simulink model "comparcion"  (R2019a)
settings: Solver=VariableStepAuto  StartTime=0.0  StopTime=10  MaxStep=1e-4  RelTol=1e-3
values from neighbouring files (symbols this model uses):
  alfa_cu = 3.9 * 10^(-3)    (= 0.0039)    [Datos.m]
  bl = 0    [Datos.m]
  bm = 1.5 * 10^(-5)    (= 1.5e-05)    [Datos.m]
  Cts = 0.818    [Datos.m]
  Jl = 0.2520    (= 0.252)    [Datos.m]
  Jm = 3.1 * 10^(-6)    (= 3.1e-06)    [Datos.m]
  lambda_m_r = 0.01546    [Datos.m]
  Ld = 6.6e-3    (= 0.0066)    [Datos.m]
  Lq = 5.8e-3    (= 0.0058)    [Datos.m]
  Pp = 3    [Datos.m]
  r = 314.3008    [Datos.m]
  Rts_amb = 146.7    [Datos.m]
undefined symbols (not defined in the file or in its folder): magnitude, sigbuilder_block
settings Model: OrderedModelArguments=off  Creator=renzo  LastModifiedBy=renzo

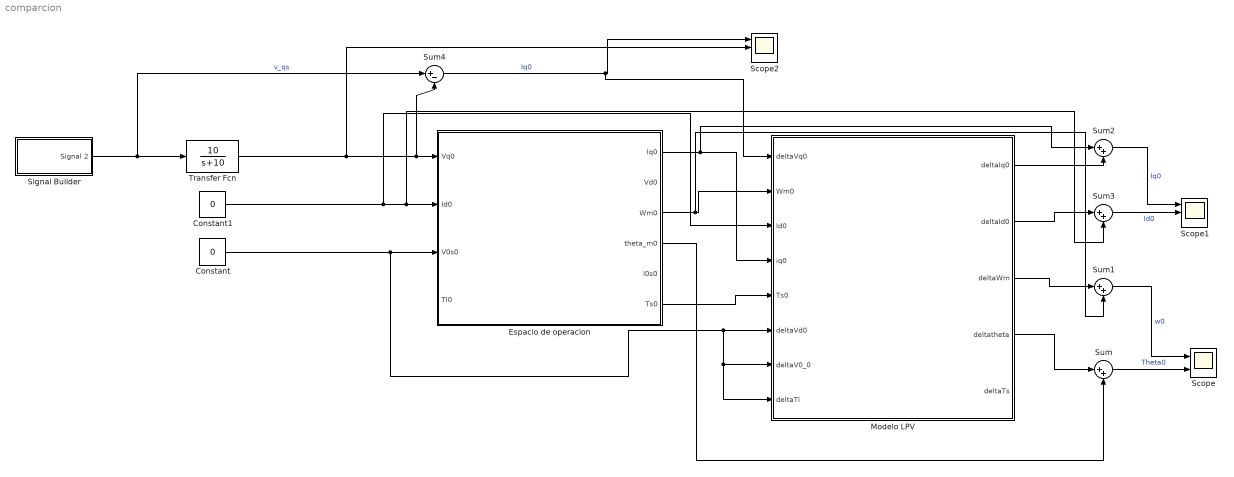
== system comparcion ==
  Constant : Constant  Value=0
  Constant1 : Constant  Value=0
  "Espacio de operacion " : Subsystem
  "Modelo LPV " : Subsystem
  Scope : Scope  NumInputPorts=2
  Scope1 : Scope  NumInputPorts=3
  Scope2 : Scope  NumInputPorts=3
  Signal Builder : Subsystem  Tag=STV Subsys  LoadFcn=sigbuilder_block('load');  StartFcn=sigbuilder_block('start');  StopFcn=sigbuilder_block('stop');  ClipboardFcn=sigbuilder_block('clipboard');  mask(Sigbuilder block){tuvar=[0:10]}
      mask help: Simulink:masks:SigbuilderBlock_MD
      mask init:
      | if ~strcmp(get_param(bdroot(gcbh),'SimulationStatus'),'stopped') tuvar = sigbuilder_block('maskInit'); end
      settings: CopyFcn=sigbuilder_block('copy');  DeleteFcn=sigbuilder_block('delete');  ModelCloseFcn=sigbuilder_block('modelClose');  PreSaveFcn=sigbuilder_block('preSave');  PauseFcn=sigbuilder_block('pause');  ContinueFcn=sigbuilder_block('continue');  NameChangeFcn=sigbuilder_block('namechange');  OpenFcn=sigbuilder_block('open',[437.6 153 550.4 359.25 ]);  CloseFcn=sigbuilder_block('close');
      mask Display: plot(0, 0, 100, 100,[2, 2, 32, 32, 2], [68, 8, 8, 68, 68],[32, 2], [38, 38], [32, 19, 2],[53, 60, 44], [32, 17, 17, 2],[16, 16, 31, 31]);txt = getActiveGroup(gcbh);text(2, 100, txt,'verticalAlignment', 'top');
  Sum{,1..3} (4 alike) : Sum  Inputs=|++
  Sum4 : Sum  Inputs=|+-
  Transfer Fcn : TransferFcn  Numerator=[10]  Denominator=[1 10]
  wires:
  Sum2/1 -> Scope1/1  "Iq0"
  Sum3/1 -> Scope1/2  "Id0"
  Transfer Fcn/1 -> Scope2/2, "Espacio de operacion "/1(Vq0), Sum4/2
  Sum4/1 -> "Modelo LPV "/1(deltaVq0), Scope2/1  "Iq0"
  Constant1/1 -> "Modelo LPV "/3(Id0), Sum3/2, "Espacio de operacion "/2(Id0)
  Constant/1 -> "Modelo LPV "/8(deltaTl), "Modelo LPV "/7("deltaV0_0 "), "Modelo LPV "/6("deltaVd0 "), "Espacio de operacion "/3(V0s0)
  "Espacio de operacion "/1(Iq0) -> Sum2/1, "Modelo LPV "/4(iq0)
  "Espacio de operacion "/3(Wm0) -> Sum1/2, "Modelo LPV "/2(Wm0)
  "Modelo LPV "/1("deltaIq0 ") -> Sum2/2
  "Modelo LPV "/2(deltaId0) -> Sum3/1
  "Modelo LPV "/3(deltaWm) -> Sum1/1
  "Espacio de operacion "/4(theta_m0) -> Sum/2
  "Modelo LPV "/4(deltatheta) -> Sum/1
  Sum1/1 -> Scope/1  "w0"
  Sum/1 -> Scope/2  "Theta0"
  Signal Builder/1(Signal 2) -> Sum4/1, Transfer Fcn/1  "v_qs"
  "Espacio de operacion "/6(Ts0) -> "Modelo LPV "/5(Ts0)

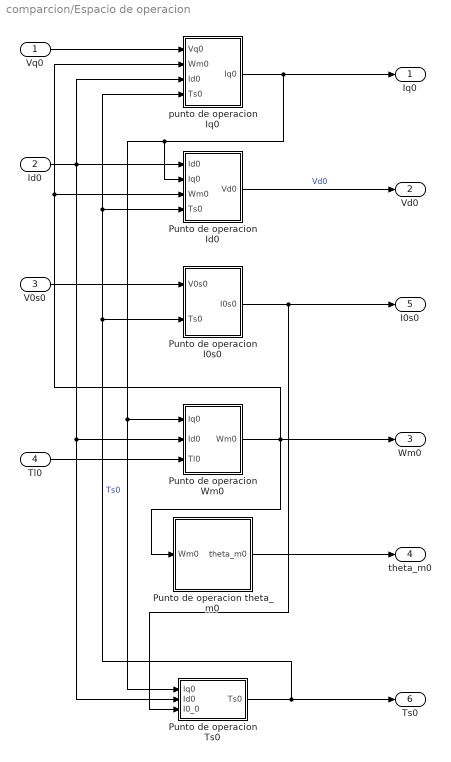
== system comparcion/Espacio de operacion  ==
  Vq0 : Inport
  Id0 : Inport  Port=2
  V0s0 : Inport  Port=3
  "Tl0 " : Inport  Port=4
  Punto de operacion I0s0 : Subsystem
  Punto de operacion Id0 : Subsystem
  Punto de operacion Ts0 : Subsystem
  Punto de operacion Wm0 : Subsystem
  Punto de operacion theta_m0 : Subsystem
  "punto de operacion Iq0 " : Subsystem
  Iq0 : Outport
  Vd0 : Outport  Port=2
  Wm0 : Outport  Port=3
  theta_m0 : Outport  Port=4
  I0s0 : Outport  Port=5
  Ts0 : Outport  Port=6
  wires:
  Punto de operacion Wm0/1("Wm0 ") -> Wm0/1, Punto de operacion Id0/3(Wm0), "punto de operacion Iq0 "/2("Wm0 "), Punto de operacion theta_m0/1(Wm0)
  Punto de operacion Ts0/1(Ts0) -> Ts0/1, Punto de operacion Id0/4("Ts0 "), "punto de operacion Iq0 "/4(Ts0), Punto de operacion I0s0/2("Ts0 ")  "Ts0"
  Punto de operacion I0s0/1("I0s0 ") -> Punto de operacion Ts0/3("I0_0 "), I0s0/1
  "punto de operacion Iq0 "/1("Iq0 ") -> Punto de operacion Id0/2("Iq0 "), Punto de operacion Wm0/1(Iq0), Punto de operacion Ts0/1(Iq0), Iq0/1
  Punto de operacion theta_m0/1("theta_m0 ") -> theta_m0/1
  Punto de operacion Id0/1("Vd0 ") -> Vd0/1  "Vd0"
  V0s0/1 -> Punto de operacion I0s0/1("V0s0 ")
  Vq0/1 -> "punto de operacion Iq0 "/1(Vq0)
  "Tl0 "/1 -> Punto de operacion Wm0/3("Tl0 ")
  Id0/1 -> Punto de operacion Ts0/2(Id0), Punto de operacion Wm0/2("Id0 "), "punto de operacion Iq0 "/3("Id0 "), Punto de operacion Id0/1("Id0 ")

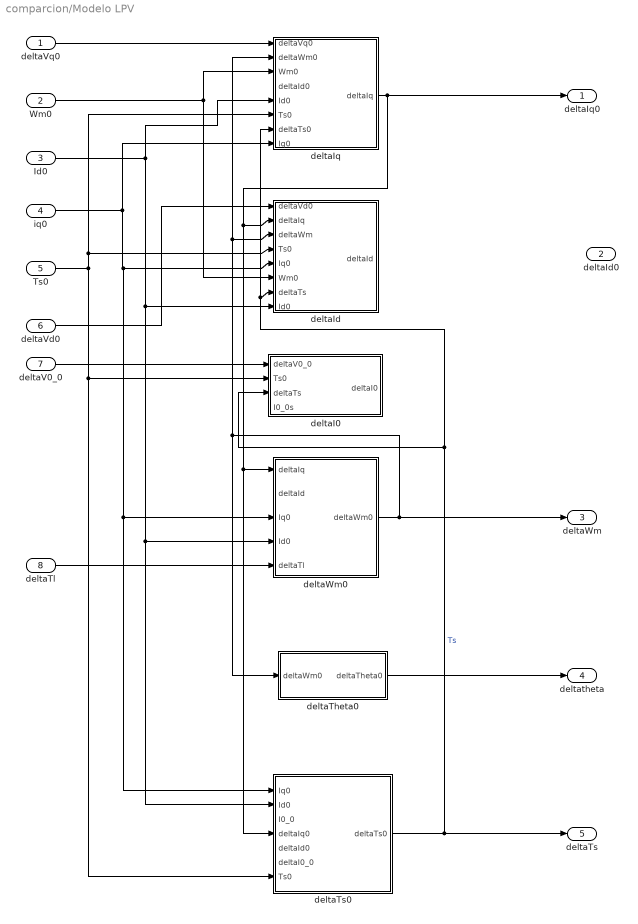
== system comparcion/Modelo LPV  ==
  deltaVq0 : Inport
  Wm0 : Inport  Port=2
  Id0 : Inport  Port=3
  iq0 : Inport  Port=4
  Ts0 : Inport  Port=5
  "deltaVd0 " : Inport  Port=6
  "deltaV0_0 " : Inport  Port=7
  deltaTl : Inport  Port=8
  deltaI0 : Subsystem
  deltaId : Subsystem
  deltaIq : Subsystem
  deltaTheta0 : Subsystem
  "deltaTs0 " : Subsystem
  deltaWm0 : Subsystem
  "deltaIq0 " : Outport
  deltaId0 : Outport  Port=2
  deltaWm : Outport  Port=3
  deltatheta : Outport  Port=4
  deltaTs : Outport  Port=5
  wires:
  "deltaTs0 "/1(deltaTs0) -> deltaTs/1, deltaIq/7("deltaTs0 "), deltaId/7(deltaTs), deltaI0/3(deltaTs)  "Ts"
  Ts0/1 -> "deltaTs0 "/7("Ts0 "), deltaI0/2("Ts0 "), deltaId/4("Ts0 "), deltaIq/6("Ts0 ")
  deltaVq0/1 -> deltaIq/1(deltaVq0)
  deltaWm0/1("deltaWm0 ") -> deltaWm/1, deltaTheta0/1("deltaWm0 "), deltaIq/2("deltaWm0 "), deltaId/3("deltaWm ")
  Wm0/1 -> deltaId/6(Wm0), deltaIq/3(Wm0)
  Id0/1 -> deltaId/8(Id0), "deltaTs0 "/2(Id0), deltaWm0/4("Id0 "), deltaIq/5(Id0)
  iq0/1 -> "deltaTs0 "/1("Iq0 "), deltaWm0/3("Iq0 "), deltaId/5(Iq0), deltaIq/8(Iq0)
  deltaIq/1(deltaIq) -> deltaWm0/1(deltaIq), "deltaTs0 "/4("deltaIq0 "), deltaId/2("deltaIq "), "deltaIq0 "/1
  "deltaVd0 "/1 -> deltaId/1(deltaVd0)
  "deltaV0_0 "/1 -> deltaI0/1(deltaV0_0)
  deltaTl/1 -> deltaWm0/5(deltaTl)
  deltaTheta0/1("deltaTheta0 ") -> deltatheta/1

== system comparcion/Signal Builder ==
  Demux : Demux  Tag=STV Demux  Outputs=1
  FromWs : FromWorkspace  Tag=STV FromWs  VariableName=tuvar  SampleTime=0
      SigBuilderData=|
      | common.afterFinalStr = 'Extrapolate'
      | common.sampleTime = 0
      | dataSet.timeRange = [0 10]
      | dataSet.name = 'Group 1'
      | sbobj.Groups.Name = 'Group 1'
      | sbobj.Groups.Signals.Name = 'Signal 2'
      | sbobj.Groups.Signals.XData = [0 1 1 10]
      | sbobj.Groups.Signals.YData = [0 0 1 1]
  Signal 2 : Outport  Tag=STV Outport
  wires:
  FromWs/1 -> Demux/1
  Demux/1 -> Signal 2/1

== system comparcion/Espacio de operacion /Punto de operacion I0s0 ==
  "V0s0 " : Inport
  "Ts0 " : Inport  Port=2
  Divide : Product  Inputs=*/
  Rs(t) : Subsystem
  "I0s0 " : Outport
  wires:
  "V0s0 "/1 -> Divide/1
  "Ts0 "/1 -> Rs(t)/1(Ts)
  Rs(t)/1(Rs) -> Divide/2
  Divide/1 -> "I0s0 "/1

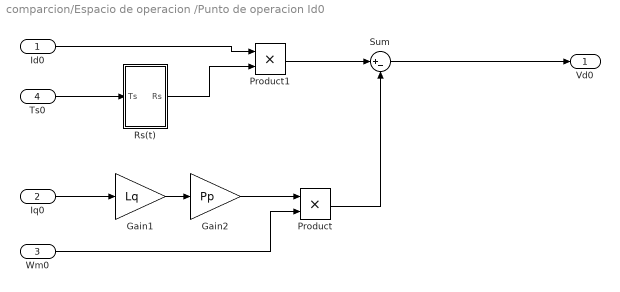
== system comparcion/Espacio de operacion /Punto de operacion Id0 ==
  "Id0 " : Inport
  "Iq0 " : Inport  Port=2
  Wm0 : Inport  Port=3
  "Ts0 " : Inport  Port=4
  Gain1 : Gain  Gain=Lq
  Gain2 : Gain  Gain=Pp
  Product : Product
  Product1 : Product
  Rs(t) : Subsystem
  Sum : Sum  Inputs=|+-
  "Vd0 " : Outport
  wires:
  "Iq0 "/1 -> Gain1/1
  Gain2/1 -> Product/1
  Gain1/1 -> Gain2/1
  Wm0/1 -> Product/2
  Product/1 -> Sum/2
  "Ts0 "/1 -> Rs(t)/1(Ts)
  Sum/1 -> "Vd0 "/1
  Rs(t)/1(Rs) -> Product1/2
  "Id0 "/1 -> Product1/1
  Product1/1 -> Sum/1

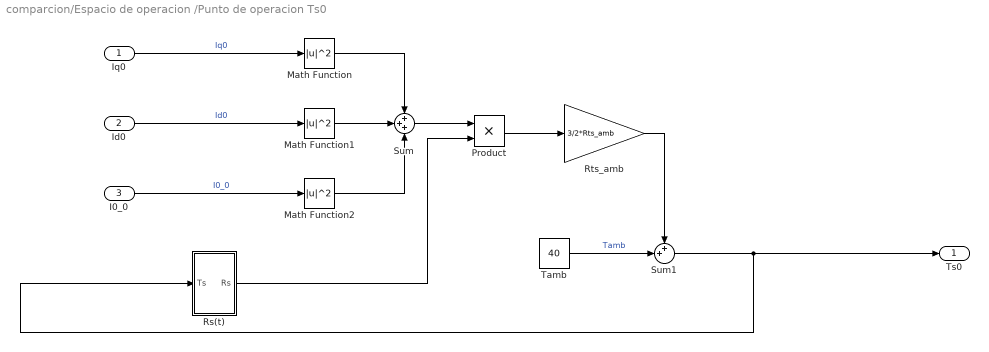
== system comparcion/Espacio de operacion /Punto de operacion Ts0 ==
  Iq0 : Inport
  Id0 : Inport  Port=2
  "I0_0 " : Inport  Port=3
  Math Function : Math  Operator=magnitude^2  SaturateOnIntegerOverflow=on
  Math Function1 : Math  Operator=magnitude^2  SaturateOnIntegerOverflow=on
  Math Function2 : Math  Operator=magnitude^2  SaturateOnIntegerOverflow=on
  Product : Product
  Rs(t) : Subsystem
  Rts_amb : Gain  Gain=3/2*Rts_amb
  Sum : Sum  Inputs=3
  Sum1 : Sum  Inputs=++|
  Tamb : Constant  Value=40
  Ts0 : Outport  VectorParamsAs1DForOutWhenUnconnected=on
  wires:
  Iq0/1 -> Math Function/1  "Iq0"
  Id0/1 -> Math Function1/1  "Id0"
  "I0_0 "/1 -> Math Function2/1  "I0_0"
  Math Function1/1 -> Sum/2
  Math Function/1 -> Sum/1
  Math Function2/1 -> Sum/3
  Sum/1 -> Product/1
  Product/1 -> Rts_amb/1
  Tamb/1 -> Sum1/2  "Tamb"
  Sum1/1 -> Ts0/1, Rs(t)/1(Ts)
  Rs(t)/1(Rs) -> Product/2
  Rts_amb/1 -> Sum1/1

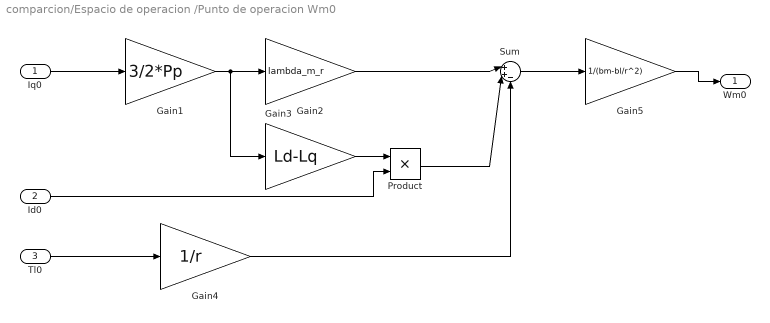
== system comparcion/Espacio de operacion /Punto de operacion Wm0 ==
  Iq0 : Inport
  "Id0 " : Inport  Port=2
  "Tl0 " : Inport  Port=3
  Gain1 : Gain  Gain=3/2*Pp
  Gain2 : Gain  Gain=lambda_m_r
  Gain3 : Gain  Gain=Ld-Lq
  Gain4 : Gain  Gain=1/r
  Gain5 : Gain  Gain=1/(bm-bl/r^2)
  Product : Product
  Sum : Sum  Inputs=|++-
  "Wm0 " : Outport
  wires:
  Iq0/1 -> Gain1/1
  Gain1/1 -> Gain3/1, Gain2/1
  Gain2/1 -> Sum/1
  Gain3/1 -> Product/1
  "Id0 "/1 -> Product/2
  Product/1 -> Sum/2
  "Tl0 "/1 -> Gain4/1
  Gain4/1 -> Sum/3
  Sum/1 -> Gain5/1
  Gain5/1 -> "Wm0 "/1

== system comparcion/Espacio de operacion /Punto de operacion theta_m0 ==
  Wm0 : Inport
  Integrator : Integrator
  "theta_m0 " : Outport
  wires:
  Wm0/1 -> Integrator/1
  Integrator/1 -> "theta_m0 "/1

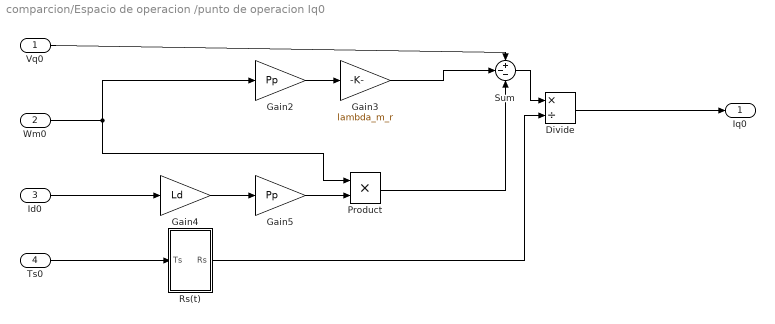
== system comparcion/Espacio de operacion /punto de operacion Iq0  ==
  Vq0 : Inport
  "Wm0 " : Inport  Port=2
  "Id0 " : Inport  Port=3
  Ts0 : Inport  Port=4
  Divide : Product  Inputs=*/
  Gain2 : Gain  Gain=Pp
  Gain3 : Gain  Gain=lambda_m_r
  Gain4 : Gain  Gain=Ld
  Gain5 : Gain  Gain=Pp
  Product : Product
  Rs(t) : Subsystem
  Sum : Sum  Inputs=+--
  "Iq0 " : Outport
  wires:
  "Wm0 "/1 -> Gain2/1, Product/1
  Gain2/1 -> Gain3/1
  Gain3/1 -> Sum/2
  Gain5/1 -> Product/2
  Gain4/1 -> Gain5/1
  "Id0 "/1 -> Gain4/1
  Product/1 -> Sum/3
  Ts0/1 -> Rs(t)/1(Ts)
  Divide/1 -> "Iq0 "/1
  Vq0/1 -> Sum/1
  Rs(t)/1(Rs) -> Divide/2
  Sum/1 -> Divide/1

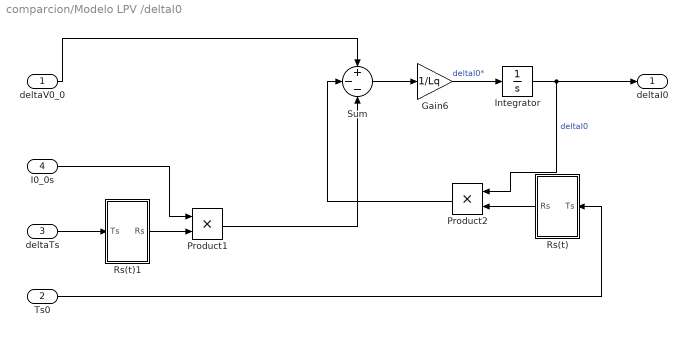
== system comparcion/Modelo LPV /deltaI0 ==
  deltaV0_0 : Inport
  "Ts0 " : Inport  Port=2
  deltaTs : Inport  Port=3
  I0_0s : Inport  Port=4
  Gain6 : Gain  Gain=1/Lq
  Integrator : Integrator
  Product1 : Product
  Product2 : Product
  Rs(t) : Subsystem
  Rs(t)1 : Subsystem
  Sum : Sum  Inputs=+--
  deltaI0 : Outport
  wires:
  deltaV0_0/1 -> Sum/1
  Sum/1 -> Gain6/1
  Gain6/1 -> Integrator/1  "deltaI0*"
  Integrator/1 -> Product2/1, deltaI0/1  "deltaI0"
  Rs(t)/1(Rs) -> Product2/2
  "Ts0 "/1 -> Rs(t)/1(Ts)
  Product2/1 -> Sum/2
  Rs(t)1/1(Rs) -> Product1/2
  deltaTs/1 -> Rs(t)1/1(Ts)
  I0_0s/1 -> Product1/1
  Product1/1 -> Sum/3

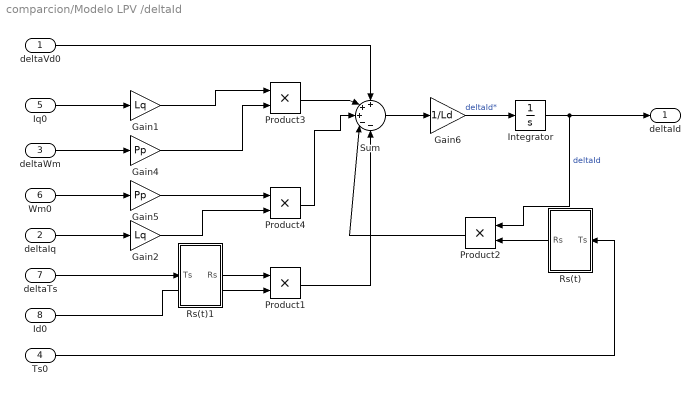
== system comparcion/Modelo LPV /deltaId ==
  deltaVd0 : Inport
  "deltaIq " : Inport  Port=2
  "deltaWm " : Inport  Port=3
  "Ts0 " : Inport  Port=4
  Iq0 : Inport  Port=5
  Wm0 : Inport  Port=6
  deltaTs : Inport  Port=7
  Id0 : Inport  Port=8
  Gain1 : Gain  Gain=Lq
  Gain2 : Gain  Gain=Lq
  Gain4 : Gain  Gain=Pp
  Gain5 : Gain  Gain=Pp
  Gain6 : Gain  Gain=1/Ld
  Integrator : Integrator
  Product{1..4} (4 alike) : Product
  Rs(t) : Subsystem
  Rs(t)1 : Subsystem
  Sum : Sum  Inputs=+++--
  deltaId : Outport
  wires:
  "deltaIq "/1 -> Gain2/1
  deltaVd0/1 -> Sum/1
  Sum/1 -> Gain6/1
  Gain6/1 -> Integrator/1  "deltaId*"
  Integrator/1 -> Product2/1, deltaId/1  "deltaId"
  Rs(t)/1(Rs) -> Product2/2
  "Ts0 "/1 -> Rs(t)/1(Ts)
  Gain1/1 -> Product3/1
  Product3/1 -> Sum/2
  "deltaWm "/1 -> Gain4/1
  Gain2/1 -> Product4/2
  Product4/1 -> Sum/3
  Product2/1 -> Sum/4
  Gain4/1 -> Product3/2
  Gain5/1 -> Product4/1
  Wm0/1 -> Gain5/1
  Rs(t)1/1(Rs) -> Product1/1
  deltaTs/1 -> Rs(t)1/1(Ts)
  Iq0/1 -> Gain1/1
  Id0/1 -> Product1/2
  Product1/1 -> Sum/5

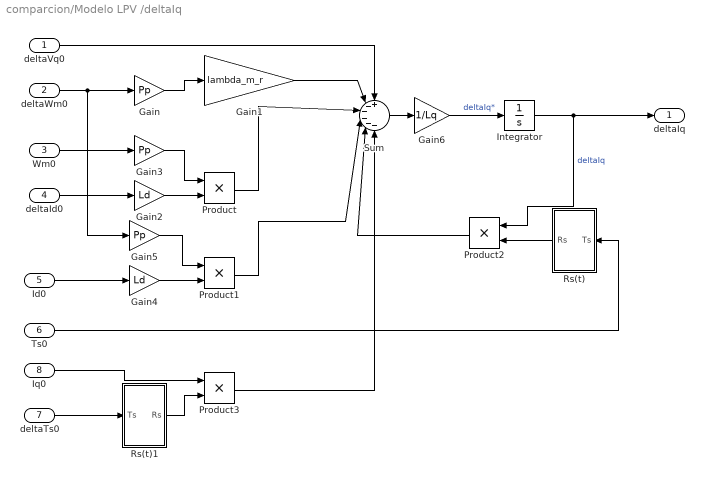
== system comparcion/Modelo LPV /deltaIq ==
  deltaVq0 : Inport
  "deltaWm0 " : Inport  Port=2
  Wm0 : Inport  Port=3
  deltaId0 : Inport  Port=4
  Id0 : Inport  Port=5
  "Ts0 " : Inport  Port=6
  "deltaTs0 " : Inport  Port=7
  Iq0 : Inport  Port=8
  Gain : Gain  Gain=Pp
  Gain1 : Gain  Gain=lambda_m_r
  Gain2 : Gain  Gain=Ld
  Gain3 : Gain  Gain=Pp
  Gain4 : Gain  Gain=Ld
  Gain5 : Gain  Gain=Pp
  Gain6 : Gain  Gain=1/Lq
  Integrator : Integrator
  Product{,1..3} (4 alike) : Product
  Rs(t) : Subsystem
  Rs(t)1 : Subsystem
  Sum : Sum  Inputs=+-----
  deltaIq : Outport
  wires:
  Gain/1 -> Gain1/1
  Gain2/1 -> Product/2
  deltaId0/1 -> Gain2/1
  deltaVq0/1 -> Sum/1
  Gain1/1 -> Sum/2
  Product/1 -> Sum/3
  Wm0/1 -> Gain3/1
  Gain3/1 -> Product/1
  "deltaWm0 "/1 -> Gain5/1, Gain/1
  Product1/1 -> Sum/4
  Gain5/1 -> Product1/1
  Gain4/1 -> Product1/2
  Id0/1 -> Gain4/1
  Sum/1 -> Gain6/1
  Gain6/1 -> Integrator/1  "deltaIq*"
  Integrator/1 -> Product2/1, deltaIq/1  "deltaIq"
  Rs(t)/1(Rs) -> Product2/2
  Product2/1 -> Sum/5
  "Ts0 "/1 -> Rs(t)/1(Ts)
  "deltaTs0 "/1 -> Rs(t)1/1(Ts)
  Rs(t)1/1(Rs) -> Product3/2
  Product3/1 -> Sum/6
  Iq0/1 -> Product3/1

== system comparcion/Modelo LPV /deltaTheta0 ==
  "deltaWm0 " : Inport
  Integrator : Integrator
  "deltaTheta0 " : Outport
  wires:
  "deltaWm0 "/1 -> Integrator/1
  Integrator/1 -> "deltaTheta0 "/1

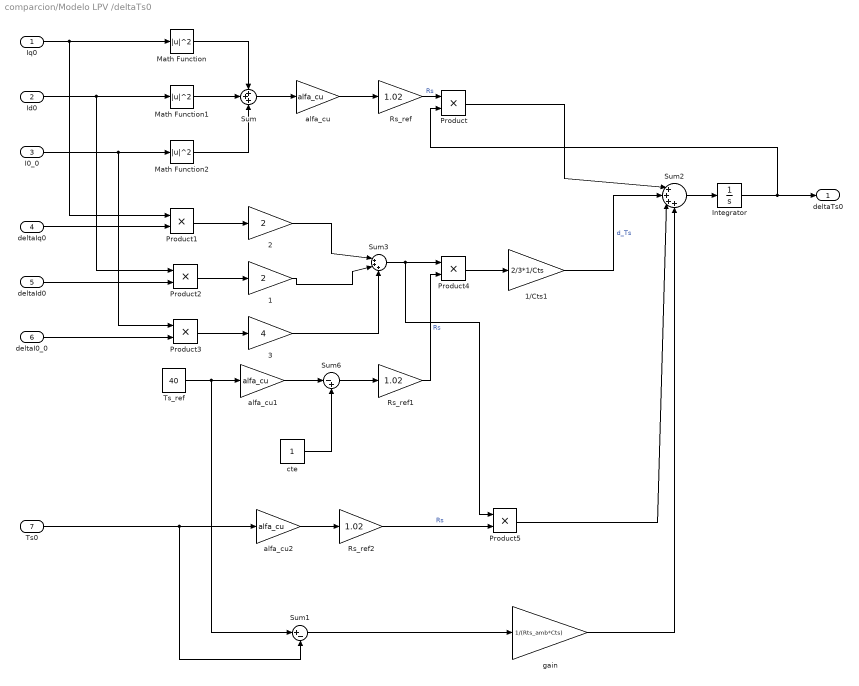
== system comparcion/Modelo LPV /deltaTs0  ==
  "Iq0 " : Inport
  Id0 : Inport  Port=2
  "I0_0 " : Inport  Port=3
  "deltaIq0 " : Inport  Port=4
  "deltaId0 " : Inport  Port=5
  deltaI0_0 : Inport  Port=6
  "Ts0 " : Inport  Port=7
  1 : Gain  Gain=2
  1/Cts1 : Gain  Gain=2/3*1/Cts
  2 : Gain  Gain=2
  3 : Gain  Gain=4
  Integrator : Integrator
  Math Function : Math  Operator=magnitude^2  SaturateOnIntegerOverflow=on
  Math Function1 : Math  Operator=magnitude^2  SaturateOnIntegerOverflow=on
  Math Function2 : Math  Operator=magnitude^2  SaturateOnIntegerOverflow=on
  Product{,1..5} (6 alike) : Product
  Rs_ref : Gain  Gain=1.02
  Rs_ref1 : Gain  Gain=1.02
  Rs_ref2 : Gain  Gain=1.02
  Sum : Sum  Inputs=3
  Sum1 : Sum  Inputs=|+-
  Sum2 : Sum  Inputs=|++++
  Sum3 : Sum  Inputs=|+++
  Sum6 : Sum  Inputs=|-+
  Ts_ref : Constant  Value=40
  alfa_cu : Gain  Gain=alfa_cu
  alfa_cu1 : Gain  Gain=alfa_cu
  alfa_cu2 : Gain  Gain=alfa_cu
  cte : Constant
  gain : Gain  Gain=1/(Rts_amb*Cts)
  deltaTs0 : Outport  VectorParamsAs1DForOutWhenUnconnected=on
  wires:
  Math Function1/1 -> Sum/2
  Math Function/1 -> Sum/1
  Math Function2/1 -> Sum/3
  "Iq0 "/1 -> Product1/1, Math Function/1
  Id0/1 -> Product2/1, Math Function1/1
  alfa_cu/1 -> Rs_ref/1
  Sum/1 -> alfa_cu/1
  Rs_ref/1 -> Product/1  "Rs"
  "deltaIq0 "/1 -> Product1/2
  deltaI0_0/1 -> Product3/2
  "deltaId0 "/1 -> Product2/2
  "I0_0 "/1 -> Product3/1, Math Function2/1
  Product1/1 -> 2/1
  Product2/1 -> 1/1
  Product3/1 -> 3/1
  2/1 -> Sum3/1
  1/1 -> Sum3/2
  3/1 -> Sum3/3
  Sum6/1 -> Rs_ref1/1
  alfa_cu1/1 -> Sum6/1
  cte/1 -> Sum6/2
  Ts_ref/1 -> Sum1/1, alfa_cu1/1
  Sum3/1 -> Product5/1, Product4/1
  Rs_ref1/1 -> Product4/2  "Rs"
  Product4/1 -> 1/Cts1/1
  alfa_cu2/1 -> Rs_ref2/1
  "Ts0 "/1 -> Sum1/2, alfa_cu2/1
  Rs_ref2/1 -> Product5/2  "Rs"
  Sum1/1 -> gain/1
  Product/1 -> Sum2/1
  1/Cts1/1 -> Sum2/2  "d_Ts"
  Product5/1 -> Sum2/3
  gain/1 -> Sum2/4
  Sum2/1 -> Integrator/1
  Integrator/1 -> Product/2, deltaTs0/1

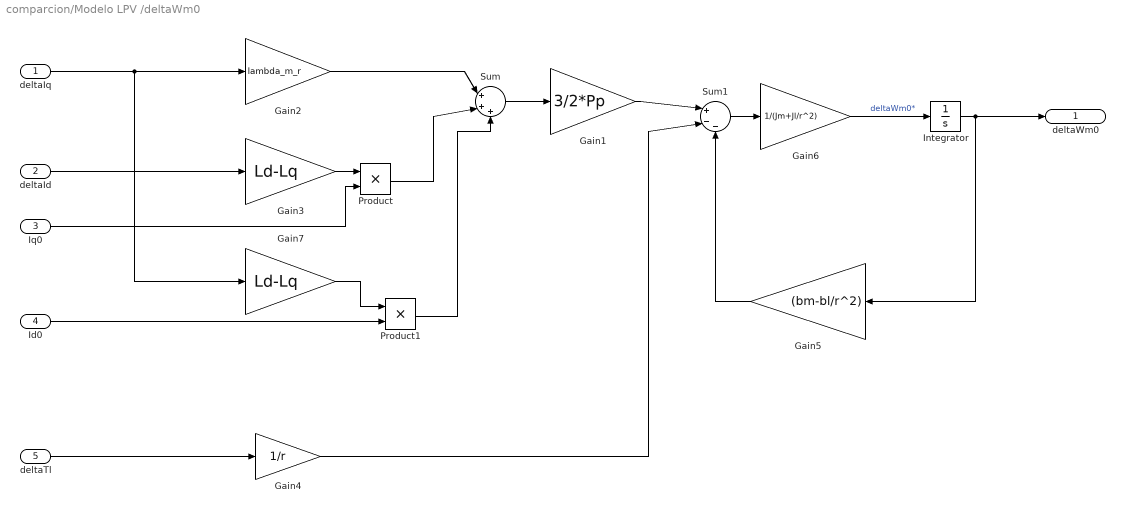
== system comparcion/Modelo LPV /deltaWm0 ==
  deltaIq : Inport
  "deltaId " : Inport  Port=2
  "Iq0 " : Inport  Port=3
  "Id0 " : Inport  Port=4
  deltaTl : Inport  Port=5
  Gain1 : Gain  Gain=3/2*Pp
  Gain2 : Gain  Gain=lambda_m_r
  Gain3 : Gain  Gain=Ld-Lq
  Gain4 : Gain  Gain=1/r
  Gain5 : Gain  Gain=(bm-bl/r^2)
  Gain6 : Gain  Gain=1/(Jm+Jl/r^2)
  Gain7 : Gain  Gain=Ld-Lq
  Integrator : Integrator
  Product : Product
  Product1 : Product
  Sum : Sum  Inputs=|+++
  Sum1 : Sum  Inputs=|+--
  "deltaWm0 " : Outport
  wires:
  Sum/1 -> Gain1/1
  deltaIq/1 -> Gain7/1, Gain2/1
  Gain2/1 -> Sum/1
  "deltaId "/1 -> Gain3/1
  Gain3/1 -> Product/1
  "Iq0 "/1 -> Product/2
  Product/1 -> Sum/2
  deltaTl/1 -> Gain4/1
  Gain7/1 -> Product1/1
  "Id0 "/1 -> Product1/2
  Product1/1 -> Sum/3
  Gain1/1 -> Sum1/1
  Gain4/1 -> Sum1/2
  Sum1/1 -> Gain6/1
  Gain5/1 -> Sum1/3
  Gain6/1 -> Integrator/1  "deltaWm0*"
  Integrator/1 -> Gain5/1, "deltaWm0 "/1

== system comparcion/Espacio de operacion /Punto de operacion I0s0/Rs(t) ==
  Ts : Inport
  Rs_ref : Gain  Gain=1.02
  Sum5 : Sum  Inputs=|+-
  Sum6 : Sum  Inputs=|++
  Ts_ref : Constant  Value=40
  alfa_cu : Gain  Gain=alfa_cu
  cte : Constant
  Rs : Outport
  wires:
  alfa_cu/1 -> Sum6/1
  Sum6/1 -> Rs_ref/1
  Rs_ref/1 -> Rs/1  "Rs"
  Ts_ref/1 -> Sum5/2
  cte/1 -> Sum6/2
  Ts/1 -> Sum5/1
  Sum5/1 -> alfa_cu/1

== system comparcion/Espacio de operacion /Punto de operacion Id0/Rs(t) ==
  Ts : Inport
  Rs_ref : Gain  Gain=1.02
  Sum5 : Sum  Inputs=|+-
  Sum6 : Sum  Inputs=|++
  Ts_ref : Constant  Value=40
  alfa_cu : Gain  Gain=alfa_cu
  cte : Constant
  Rs : Outport
  wires:
  alfa_cu/1 -> Sum6/1
  Sum6/1 -> Rs_ref/1
  Rs_ref/1 -> Rs/1  "Rs"
  Ts_ref/1 -> Sum5/2
  cte/1 -> Sum6/2
  Ts/1 -> Sum5/1
  Sum5/1 -> alfa_cu/1

== system comparcion/Espacio de operacion /Punto de operacion Ts0/Rs(t) ==
  Ts : Inport
  Rs_ref : Gain  Gain=1.02
  Sum5 : Sum  Inputs=|+-
  Sum6 : Sum  Inputs=|++
  Ts_ref : Constant  Value=40
  alfa_cu : Gain  Gain=alfa_cu
  cte : Constant
  Rs : Outport
  wires:
  alfa_cu/1 -> Sum6/1
  Sum6/1 -> Rs_ref/1
  Rs_ref/1 -> Rs/1  "Rs"
  Ts_ref/1 -> Sum5/2
  cte/1 -> Sum6/2
  Ts/1 -> Sum5/1
  Sum5/1 -> alfa_cu/1

== system comparcion/Espacio de operacion /punto de operacion Iq0 /Rs(t) ==
  Ts : Inport
  Rs_ref : Gain  Gain=1.02
  Sum5 : Sum  Inputs=|+-
  Sum6 : Sum  Inputs=|++
  Ts_ref : Constant  Value=40
  alfa_cu : Gain  Gain=alfa_cu
  cte : Constant
  Rs : Outport
  wires:
  alfa_cu/1 -> Sum6/1
  Sum6/1 -> Rs_ref/1
  Rs_ref/1 -> Rs/1  "Rs"
  Ts_ref/1 -> Sum5/2
  cte/1 -> Sum6/2
  Ts/1 -> Sum5/1
  Sum5/1 -> alfa_cu/1

== system comparcion/Modelo LPV /deltaI0/Rs(t) ==
  Ts : Inport
  Rs_ref : Gain  Gain=1.02
  Sum5 : Sum  Inputs=|+-
  Sum6 : Sum  Inputs=|++
  Ts_ref : Constant  Value=40
  alfa_cu : Gain  Gain=alfa_cu
  cte : Constant
  Rs : Outport
  wires:
  alfa_cu/1 -> Sum6/1
  Sum6/1 -> Rs_ref/1
  Rs_ref/1 -> Rs/1  "Rs"
  Ts_ref/1 -> Sum5/2
  cte/1 -> Sum6/2
  Ts/1 -> Sum5/1
  Sum5/1 -> alfa_cu/1

== system comparcion/Modelo LPV /deltaI0/Rs(t)1 ==
  Ts : Inport
  Rs_ref : Gain  Gain=1.02
  Sum5 : Sum  Inputs=|+-
  Sum6 : Sum  Inputs=|++
  Ts_ref : Constant  Value=40
  alfa_cu : Gain  Gain=alfa_cu
  cte : Constant
  Rs : Outport
  wires:
  alfa_cu/1 -> Sum6/1
  Sum6/1 -> Rs_ref/1
  Rs_ref/1 -> Rs/1  "Rs"
  Ts_ref/1 -> Sum5/2
  cte/1 -> Sum6/2
  Ts/1 -> Sum5/1
  Sum5/1 -> alfa_cu/1

== system comparcion/Modelo LPV /deltaId/Rs(t) ==
  Ts : Inport
  Rs_ref : Gain  Gain=1.02
  Sum5 : Sum  Inputs=|+-
  Sum6 : Sum  Inputs=|++
  Ts_ref : Constant  Value=40
  alfa_cu : Gain  Gain=alfa_cu
  cte : Constant
  Rs : Outport
  wires:
  alfa_cu/1 -> Sum6/1
  Sum6/1 -> Rs_ref/1
  Rs_ref/1 -> Rs/1  "Rs"
  Ts_ref/1 -> Sum5/2
  cte/1 -> Sum6/2
  Ts/1 -> Sum5/1
  Sum5/1 -> alfa_cu/1

== system comparcion/Modelo LPV /deltaId/Rs(t)1 ==
  Ts : Inport
  Rs_ref : Gain  Gain=1.02
  Sum5 : Sum  Inputs=|+-
  Sum6 : Sum  Inputs=|++
  Ts_ref : Constant  Value=40
  alfa_cu : Gain  Gain=alfa_cu
  cte : Constant
  Rs : Outport
  wires:
  alfa_cu/1 -> Sum6/1
  Sum6/1 -> Rs_ref/1
  Rs_ref/1 -> Rs/1  "Rs"
  Ts_ref/1 -> Sum5/2
  cte/1 -> Sum6/2
  Ts/1 -> Sum5/1
  Sum5/1 -> alfa_cu/1

== system comparcion/Modelo LPV /deltaIq/Rs(t) ==
  Ts : Inport
  Rs_ref : Gain  Gain=1.02
  Sum5 : Sum  Inputs=|+-
  Sum6 : Sum  Inputs=|++
  Ts_ref : Constant  Value=40
  alfa_cu : Gain  Gain=alfa_cu
  cte : Constant
  Rs : Outport
  wires:
  alfa_cu/1 -> Sum6/1
  Sum6/1 -> Rs_ref/1
  Rs_ref/1 -> Rs/1  "Rs"
  Ts_ref/1 -> Sum5/2
  cte/1 -> Sum6/2
  Ts/1 -> Sum5/1
  Sum5/1 -> alfa_cu/1

== system comparcion/Modelo LPV /deltaIq/Rs(t)1 ==
  Ts : Inport
  Rs_ref : Gain  Gain=1.02
  Sum5 : Sum  Inputs=|+-
  Sum6 : Sum  Inputs=|++
  Ts_ref : Constant  Value=40
  alfa_cu : Gain  Gain=alfa_cu
  cte : Constant
  Rs : Outport
  wires:
  alfa_cu/1 -> Sum6/1
  Sum6/1 -> Rs_ref/1
  Rs_ref/1 -> Rs/1  "Rs"
  Ts_ref/1 -> Sum5/2
  cte/1 -> Sum6/2
  Ts/1 -> Sum5/1
  Sum5/1 -> alfa_cu/1
